simulink model "full_sim"  (R2021b)
settings: Solver=FixedStepAuto  StartTime=400  StopTime=1400  FixedStep=1  RelTol=1e-3
undefined symbols (not defined in the file or in its folder): A_G, G0, Gb, Ib, Vg, X0
settings Model: Creator=marek  LastModifiedBy=marekwadinger
settings DataIOCC: ExternalInput=tt

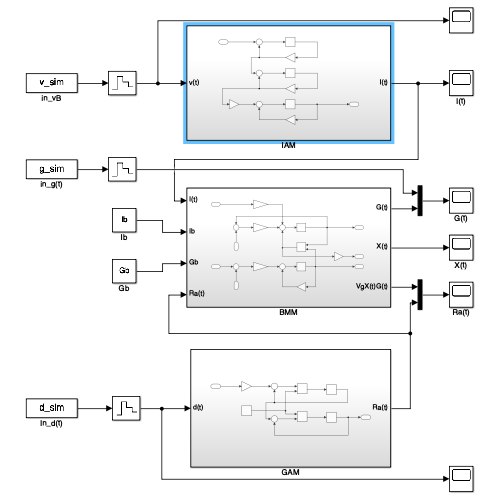
[thumbnail: Simulink's stored preview of the top-level diagram]
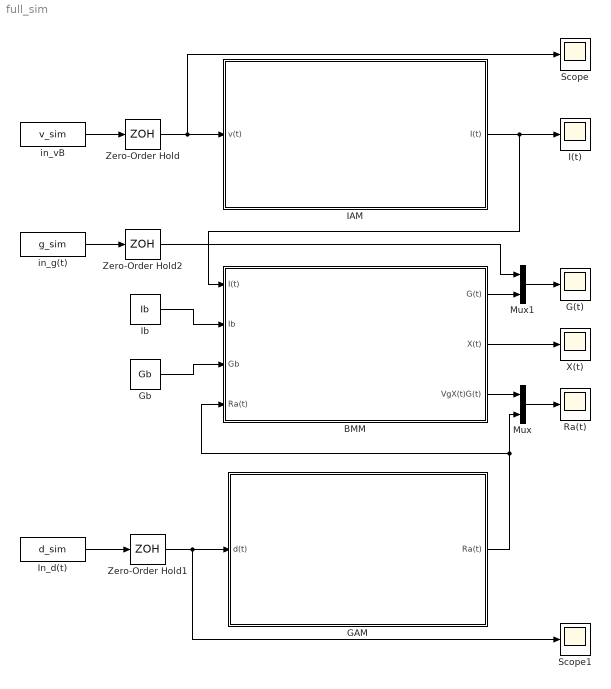
== system full_sim ==
  BMM : Subsystem
  G(t) : Scope
  GAM : Subsystem
  Gb : Constant  Value=Gb  SampleTime=0
  I(t) : Scope
  IAM : Subsystem
  Ib : Constant  Value=Ib  SampleTime=0
  In_d(t) : FromWorkspace  VariableName=d_sim
  Mux : Mux  Inputs=2
  Mux1 : Mux  Inputs=2
  Ra(t) : Scope
  Scope : Scope
  Scope1 : Scope
  X(t) : Scope
  Zero-Order Hold : ZeroOrderHold  SampleTime=-1
  Zero-Order Hold1 : ZeroOrderHold  SampleTime=-1
  Zero-Order Hold2 : ZeroOrderHold  SampleTime=-1
  in_g(t) : FromWorkspace  VariableName=g_sim
  in_vB : FromWorkspace  VariableName=v_sim
  wires:
  BMM/2(X(t)) -> X(t)/1
  BMM/1(G(t)) -> Mux1/2
  IAM/1(I(t)) -> BMM/1(I(t)), I(t)/1
  Zero-Order Hold/1 -> IAM/1(v(t)), Scope/1
  BMM/3(VgX(t)G(t)) -> Mux/1
  Mux/1 -> Ra(t)/1
  In_d(t)/1 -> Zero-Order Hold1/1
  GAM/1(Ra(t)) -> BMM/4(Ra(t)), Mux/2
  Mux1/1 -> G(t)/1
  in_g(t)/1 -> Zero-Order Hold2/1
  in_vB/1 -> Zero-Order Hold/1
  Zero-Order Hold1/1 -> Scope1/1, GAM/1(d(t))
  Zero-Order Hold2/1 -> Mux1/1
  Ib/1 -> BMM/2(Ib)
  Gb/1 -> BMM/3(Gb)

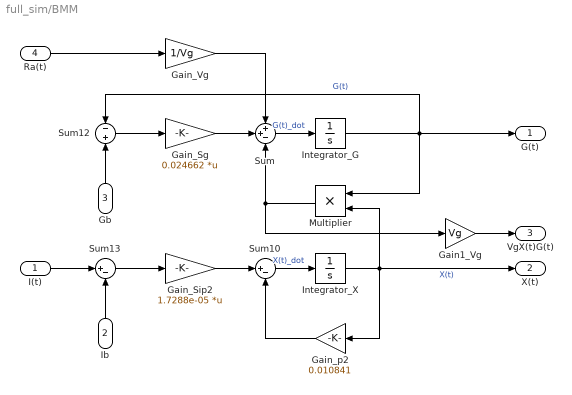
== system full_sim/BMM ==
  I(t) : Inport
  Ib : Inport  Port=2
  Gb : Inport  Port=3
  Ra(t) : Inport  Port=4
  Gain1_Vg : Gain  Gain=Vg
  Gain_Sg : Gain  Gain=0.024662  Multiplication=Matrix(K*u)
  Gain_Sip2 : Gain  Gain=1.7288e-05  Multiplication=Matrix(K*u)
  Gain_Vg : Gain  Gain=1/Vg
  Gain_p2 : Gain  Gain=0.010841
  Integrator_G : Integrator  InitialCondition=G0  UpperSaturationLimit=100  LowerSaturationLimit=0
  Integrator_X : Integrator  InitialCondition=X0
  Multiplier : Product
  Sum : Sum  Inputs=++-
  Sum10 : Sum  Inputs=|+-
  Sum12 : Sum  Inputs=-|+
  Sum13 : Sum  Inputs=|+-
  G(t) : Outport
  X(t) : Outport  Port=2
  VgX(t)G(t) : Outport  Port=3
  wires:
  Sum13/1 -> Gain_Sip2/1
  Integrator_X/1 -> Gain_p2/1, X(t)/1, Multiplier/2  "X(t)"
  Integrator_G/1 -> Multiplier/1, G(t)/1, Sum12/1  "G(t)"
  Gb/1 -> Sum12/2
  Multiplier/1 -> Sum/3, Gain1_Vg/1
  I(t)/1 -> Sum13/1
  Sum10/1 -> Integrator_X/1  "X(t)_dot"
  Ib/1 -> Sum13/2
  Sum12/1 -> Gain_Sg/1
  Sum/1 -> Integrator_G/1  "G(t)_dot"
  Gain_p2/1 -> Sum10/2
  Gain_Vg/1 -> Sum/1
  Gain_Sip2/1 -> Sum10/1
  Gain_Sg/1 -> Sum/2
  Ra(t)/1 -> Gain_Vg/1
  Gain1_Vg/1 -> VgX(t)G(t)/1

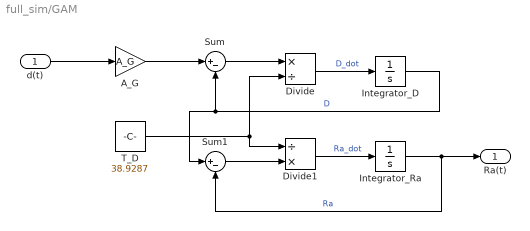
== system full_sim/GAM ==
  d(t) : Inport
  A_G : Gain  Gain=A_G
  Divide : Product  Inputs=*/
  Divide1 : Product  Inputs=/*
  Integrator_D : Integrator
  Integrator_Ra : Integrator
  Sum : Sum  Inputs=|+-
  Sum1 : Sum  Inputs=|+-
  T_D : Constant  Value=38.9287
  Ra(t) : Outport
  wires:
  Sum/1 -> Divide/1
  Divide/1 -> Integrator_D/1  "D_dot"
  Integrator_D/1 -> Sum1/1, Sum/2  "D"
  Sum1/1 -> Divide1/2
  Divide1/1 -> Integrator_Ra/1  "Ra_dot"
  A_G/1 -> Sum/1
  Integrator_Ra/1 -> Ra(t)/1, Sum1/2  "Ra"
  d(t)/1 -> A_G/1
  T_D/1 -> Divide1/1, Divide/2

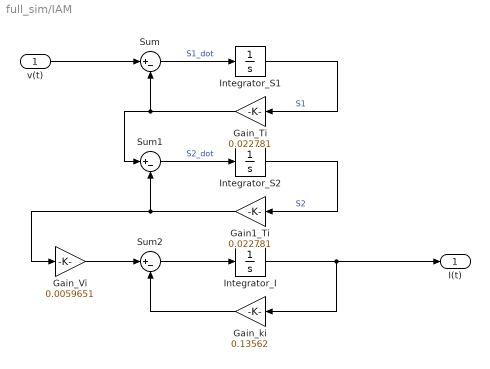
== system full_sim/IAM ==
  v(t) : Inport
  Gain1_Ti : Gain  Gain=0.022781
  Gain_Ti : Gain  Gain=0.022781
  Gain_Vi : Gain  Gain=0.0059651
  Gain_ki : Gain  Gain=0.13562
  Integrator_I : Integrator  InitialCondition=12.3686  LimitOutput=on  UpperSaturationLimit=1000  LowerSaturationLimit=0
  Integrator_S1 : Integrator  InitialCondition=12344.6425
  Integrator_S2 : Integrator  InitialCondition=12344.6425
  Sum : Sum  Inputs=|+-
  Sum1 : Sum  Inputs=|+-
  Sum2 : Sum  Inputs=|+-
  I(t) : Outport
  wires:
  Integrator_S2/1 -> Gain1_Ti/1  "S2"
  Integrator_I/1 -> I(t)/1, Gain_ki/1
  Sum2/1 -> Integrator_I/1
  Sum1/1 -> Integrator_S2/1  "S2_dot"
  Gain1_Ti/1 -> Gain_Vi/1, Sum1/2
  Sum/1 -> Integrator_S1/1  "S1_dot"
  v(t)/1 -> Sum/1
  Gain_ki/1 -> Sum2/2
  Integrator_S1/1 -> Gain_Ti/1  "S1"
  Gain_Vi/1 -> Sum2/1
  Gain_Ti/1 -> Sum1/1, Sum/2
